simulink library "Lib_PFSys_NewGenericMotor_TMATS"  (R2019b)
settings: Solver=ode45  StartTime=0.0  StopTime=10.0  RelTol=1e-3  EnableMultiTasking=on
Description:
  | Thomas Modules
settings Model: Creator=jwchapm2  LastModifiedBy=mebell
settings DataIOCC: LimitDataPoints=on  SaveFormat=Array  ReturnWorkspaceOutputs=off
settings OptimizationCC: ExpressionDepthLimit=2147483647  LifeSpan=inf
settings DebuggingCC: UnderspecifiedInitializationDetection=Classic  MergeDetectMultiDrivingBlocksExec=none  SolverPrmCheckMsg=warning  StateNameClashWarn=warning  SFUnexpectedBacktrackingDiag=warning  SFNoUnconditionalDefaultTransitionDiag=warning  SFExecutionAtInitializationDiag=none  ArithmeticOperatorsInVariantConditions=warning
settings HardwareCC: ProdBitPerPointer=32  ProdBitPerSizeT=32  ProdBitPerPtrDiffT=32  ProdLargestAtomicFloat=None  ProdIntDivRoundTo=Undefined  ProdEndianess=Unspecified  ProdWordSize=32  ProdHWDeviceType=32-bit Generic
settings ModelReferenceCC: PropagateSignalLabelsOutOfModel=off
settings SFSimCC: SimUseLocalCustomCode=off  CustomCodeUndefinedFunction=UseInterfaceOnly
settings RTWCC: RTWUseLocalCustomCode=off
settings CodeAppCC: StateflowObjectComments=on
settings GRTTargetCC: TargetLangStandard=C89/C90 (ANSI)  GeneratePreprocessorConditionals=Disable all
settings ConfigComp: CovMetricSettings=dw  CovHtmlReporting=on  CovSaveCumulativeToWorkspaceVar=on  CovSaveSingleToWorkspaceVar=on  CovExternalEMLEnable=off

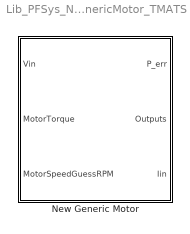
== system Lib_PFSys_NewGenericMotor_TMATS ==
  New Generic Motor : Subsystem  mask(Motor){X_C_SpeedVec_M=[0.0 0.1 1.0], Y_C_TorqueVec_M=[0.0 0.1 1.0], T_C_EffArray_M=[0.5 0.5 0.5; 0.5 1.0 1.0; 0.5 1.0 1.0], Z_M=0.01}
      mask prompts: X_C_SpeedVec_M "X_C_SpeedVec_M - Efficiency Table Speed Vector (X-axis)(nx1)"; Y_C_TorqueVec_M "Y_C_TorqueVec_M - Efficiency Table Torque Vector (Y-axis)(mx1)"; T_C_EffArray_M "T_C_EffArray_M - Efficiency Table Values (Eff = f(i, V)(nxm)"; Z_M "Z_M - Resistive Impedance"
      mask help:
      | This block represents a generic motor with a purely resistive input
      | impedance, and a lumped efficiency/loss model, specified as a lookup table.

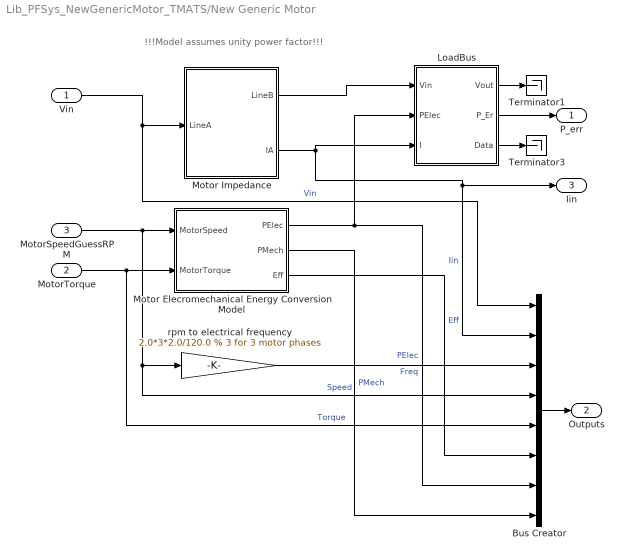
== system Lib_PFSys_NewGenericMotor_TMATS/New Generic Motor ==
  note: !!!Model assumes unity power factor!!!
  Vin : Inport
  MotorTorque : Inport  Port=2
  MotorSpeedGuessRPM : Inport  Port=3
  Bus Creator : BusCreator  Inputs=8
  LoadBus : Subsystem  AncestorBlock=Lib_PF_BusLoadDC_TMATS/LoadBus DC  mask{PeInEN_M=on, P_M=-2, BlkNm_M=double(gcb)}
      mask prompts: PeInEN_M "PeInEN_M - External Pelec"; P_M "P_M - Real power"; BlkNm_M "Block name as double for simulink output"
      mask init:
      | %Manage Power Inputs
      | if PeInEN_M == 1
      |     if strcmp(get_param([BlkNm_M '/Pelec'],'BlockType'),'Constant')
      |         MSK_ReplaceBlock_TMATS([BlkNm_M '/Pelec'],'built-in/Inport');
      |     end
      |     set_param([BlkNm_M '/Pelec'],'Port',num2str(2));
      | elseif PeInEN_M == 0
      |     if strcmp(get_param([BlkNm_M '/Pelec'],'BlockType'),'Inport')
      |         MSK_ReplaceBlock_TMATS([BlkNm_M '/Pelec'],'built-in/Constant');
      |         set_param([BlkNm_M '/Pelec'],'Value','P_M');
      |     end
      | end
      mask Callback PeInEN_M: MSK_SEC_Enables_TMATS('PeInEN_M',2,'dis')
  Motor Elecromechanical Energy Conversion Model : Subsystem
  Motor Impedance : Subsystem  AncestorBlock=Lib_PF_LineDC_TMATS/Line DC  mask{R_M=Z_M}
      mask prompts: R_M "R_M - Z Resistance"
      mask Display:
      | fprintf('R: %g',R_M)
      | port_label('input',1,'VA')
      | port_label('output',1,'VA')
      | port_label('output',2,'IA')
  Terminator1 : Terminator
  Terminator3 : Terminator
  rpm to electrical frequency : Gain  Gain=2.0*3*2.0/120.0 % 3 for 3 motor phases
  P_err : Outport  VectorParamsAs1DForOutWhenUnconnected=off
  Outputs : Outport  Port=2  VectorParamsAs1DForOutWhenUnconnected=off
  Iin : Outport  Port=3  VectorParamsAs1DForOutWhenUnconnected=off
  wires:
  Motor Elecromechanical Energy Conversion Model/1(PElec) -> LoadBus/2("PElec "), Bus Creator/7  "PElec"
  Motor Impedance/2(IA) -> Iin/1, Bus Creator/2, LoadBus/3(I)  "Iin"
  Motor Impedance/1(LineB) -> LoadBus/1(Vin)
  Bus Creator/1 -> Outputs/1
  rpm to electrical frequency/1 -> Bus Creator/3  "Freq"
  MotorTorque/1 -> Bus Creator/5, Motor Elecromechanical Energy Conversion Model/2(MotorTorque)  "Torque"
  MotorSpeedGuessRPM/1 -> Motor Elecromechanical Energy Conversion Model/1(MotorSpeed), Bus Creator/4, rpm to electrical frequency/1  "Speed"
  LoadBus/3(Data) -> Terminator3/1
  Vin/1 -> Bus Creator/1, Motor Impedance/1(LineA)  "Vin"
  LoadBus/2(P_Er) -> P_err/1
  LoadBus/1(Vout) -> Terminator1/1
  Motor Elecromechanical Energy Conversion Model/3(Eff) -> Bus Creator/6  "Eff"
  Motor Elecromechanical Energy Conversion Model/2(PMech) -> Bus Creator/8  "PMech"

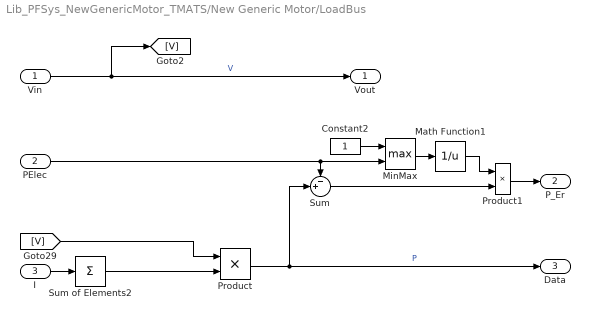
== system Lib_PFSys_NewGenericMotor_TMATS/New Generic Motor/LoadBus ==
  Vin : Inport
  "PElec " : Inport  Port=2
  I : Inport  Port=3
  Constant2 : Constant
  Math Function1 : Math  Operator=reciprocal  SaturateOnIntegerOverflow=on
  MinMax : MinMax  Function=max  Inputs=2
  Product : Product
  Product1 : Product
  Sum : Sum  Inputs=-+|
  Sum of Elements2 : Sum  Inputs=+
  Vout : Outport
  P_Er : Outport  Port=2
  Data : Outport  Port=3
  wires:
  Sum/1 -> Product1/2
  Product1/1 -> P_Er/1
  Math Function1/1 -> Product1/1
  MinMax/1 -> Math Function1/1
  Constant2/1 -> MinMax/1
  "PElec "/1 -> Sum/1, MinMax/2
  Vin/1 -> [V], Vout/1  "V"
  Product/1 -> Sum/2, Data/1  "P"
  I/1 -> Sum of Elements2/1
  [V] -> Product/1
  Sum of Elements2/1 -> Product/2

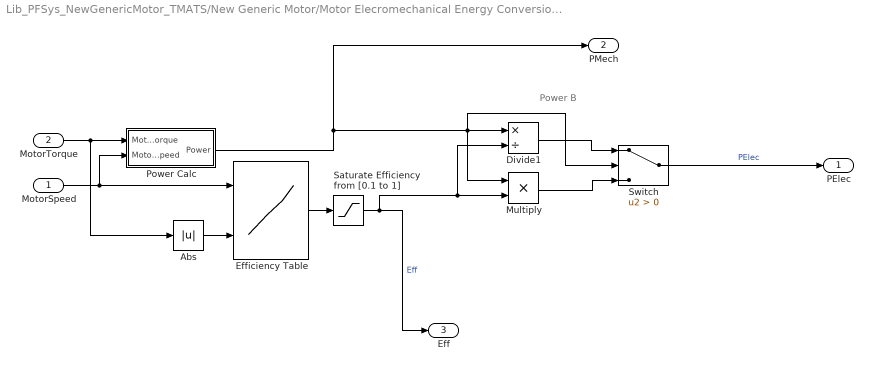
== system Lib_PFSys_NewGenericMotor_TMATS/New Generic Motor/Motor Elecromechanical Energy Conversion Model ==
  note: Power B
  MotorSpeed : Inport
  MotorTorque : Inport  Port=2
  Abs : Abs
  Divide1 : Product  Inputs=*/
  Efficiency Table : Lookup_n-D  BreakpointsForDimension1=X_C_SpeedVec_M  BreakpointsForDimension2=Y_C_TorqueVec_M  Table=T_C_EffArray_M  ExtrapMethod=Clip  InternalRulePriority=Speed  RndMeth=Simplest  InputSameDT=on
  Multiply : Product
  Power Calc : Subsystem
  Saturate Efficiency from [0.1 to 1] : Saturate  UpperLimit=1  LowerLimit=0.1
  Switch : Switch  Criteria=u2 > Threshold
  PElec : Outport  VectorParamsAs1DForOutWhenUnconnected=off
  PMech : Outport  Port=2  VectorParamsAs1DForOutWhenUnconnected=off
  Eff : Outport  Port=3  VectorParamsAs1DForOutWhenUnconnected=off
  wires:
  Efficiency Table/1 -> Saturate Efficiency from [0.1 to 1]/1
  Saturate Efficiency from [0.1 to 1]/1 -> Divide1/2, Multiply/2, Eff/1  "Eff"
  Abs/1 -> Efficiency Table/2
  Switch/1 -> PElec/1  "PElec"
  MotorTorque/1 -> Abs/1, Power Calc/1(MotorTorque)
  MotorSpeed/1 -> Power Calc/2(MotorSpeed), Efficiency Table/1
  Power Calc/1(Power) -> Switch/2, Multiply/1, Divide1/1, PMech/1
  Divide1/1 -> Switch/1
  Multiply/1 -> Switch/3

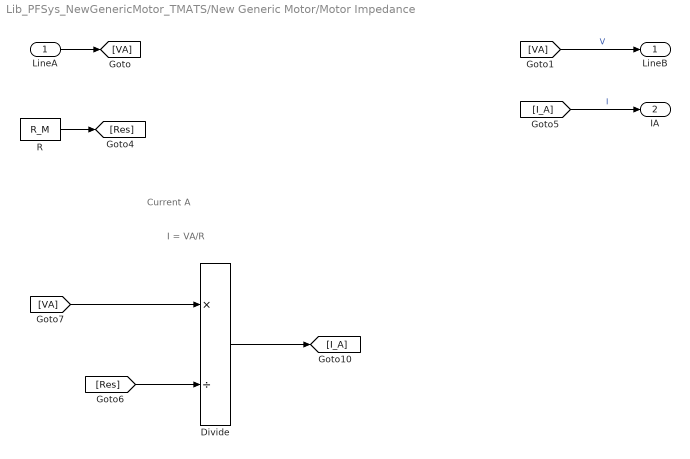
== system Lib_PFSys_NewGenericMotor_TMATS/New Generic Motor/Motor Impedance ==
  note: Current A
  note: I = VA/R
  LineA : Inport
  Divide : Product  Inputs=*/
  R : Constant  Value=R_M
  LineB : Outport
  IA : Outport  Port=2
  wires:
  [Res] -> Divide/2
  Divide/1 -> [I_A]
  [VA] -> Divide/1
  R/1 -> [Res]
  [VA] -> LineB/1  "V"
  [I_A] -> IA/1  "I"
  LineA/1 -> [VA]

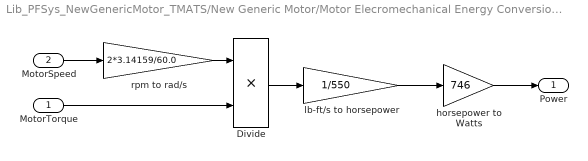
== system Lib_PFSys_NewGenericMotor_TMATS/New Generic Motor/Motor Elecromechanical Energy Conversion Model/Power Calc ==
  MotorTorque : Inport
  MotorSpeed : Inport  Port=2
  Divide : Product  Inputs=**
  horsepower to Watts : Gain  Gain=746
  lb-ft/s to horsepower : Gain  Gain=1/550
  rpm to rad/s : Gain  Gain=2*3.14159/60.0
  Power : Outport  VectorParamsAs1DForOutWhenUnconnected=off
  wires:
  MotorSpeed/1 -> rpm to rad/s/1
  Divide/1 -> lb-ft/s to horsepower/1
  lb-ft/s to horsepower/1 -> horsepower to Watts/1
  MotorTorque/1 -> Divide/2
  rpm to rad/s/1 -> Divide/1
  horsepower to Watts/1 -> Power/1
